simulink model "BallastSystemArchitecture"  (R2026a)
settings: Solver=VariableStepAuto
model workspace (MAT data in the model file):
  Control_Interface = Simulink.Bus
  Control_Interface.Alignment = -1
  Control_Interface.PreserveElementDimensions = 0
  Control_Interface.Elements_internal(1) = Simulink.BusElement
  Control_Interface.Elements_internal(1).Min_internal = 0
  Control_Interface.Elements_internal(1).Max_internal = 100
  Control_Interface.Elements_internal(1).DimensionsMode = 'Fixed'
  Control_Interface.Elements_internal(1).SamplingMode = 'Sample based'
  Control_Interface.Elements_internal(1).SampleTime = -1
  Control_Interface.Elements_internal(1).DocUnits = '%'
  Control_Interface.Elements_internal(1).Name = 'TankLevel'
  Control_Interface.Elements_internal(1).DataType_internal = 'double'
  Control_Interface.Elements_internal(1).Complexity = 'real'
  Control_Interface.Elements_internal(1).Dimensions = 1
  Control_Interface.Elements_internal(2) = Simulink.BusElement
  Control_Interface.Elements_internal(2).Min_internal = 0
  Control_Interface.Elements_internal(2).Max_internal = 1800
  Control_Interface.Elements_internal(2).DimensionsMode = 'Fixed'
  Control_Interface.Elements_internal(2).SamplingMode = 'Sample based'
  Control_Interface.Elements_internal(2).SampleTime = -1
  Control_Interface.Elements_internal(2).DocUnits = 'rpm'
  Control_Interface.Elements_internal(2).Name = 'PumpSpeed'
  Control_Interface.Elements_internal(2).DataType_internal = 'double'
  Control_Interface.Elements_internal(2).Complexity = 'real'
  Control_Interface.Elements_internal(2).Dimensions = 1
  Control_Interface.Elements_internal(3) = Simulink.BusElement
  Control_Interface.Elements_internal(3).Min_internal = 0
  Control_Interface.Elements_internal(3).Max_internal = 1
  Control_Interface.Elements_internal(3).DimensionsMode = 'Fixed'
  Control_Interface.Elements_internal(3).SamplingMode = 'Sample based'
  Control_Interface.Elements_internal(3).SampleTime = -1
  Control_Interface.Elements_internal(3).Name = 'ValveCommand'
  Control_Interface.Elements_internal(3).DataType_internal = 'boolean'
  Control_Interface.Elements_internal(3).Complexity = 'real'
  Control_Interface.Elements_internal(3).Dimensions = 1
  Control_Interface.DataScope = 'Auto'
  Electrical_Interface = Simulink.Bus
  Electrical_Interface.Alignment = -1
  Electrical_Interface.PreserveElementDimensions = 0
  Electrical_Interface.Elements_internal(1) = Simulink.BusElement
  Electrical_Interface.Elements_internal(1).Min_internal = 0
  Electrical_Interface.Elements_internal(1).Max_internal = 135
  Electrical_Interface.Elements_internal(1).DimensionsMode = 'Fixed'
  Electrical_Interface.Elements_internal(1).SamplingMode = 'Sample based'
  Electrical_Interface.Elements_internal(1).SampleTime = -1
  Electrical_Interface.Elements_internal(1).DocUnits = 'hp'
  Electrical_Interface.Elements_internal(1).Name = 'PowerDemand'
  Electrical_Interface.Elements_internal(1).DataType_internal = 'double'
  Electrical_Interface.Elements_internal(1).Complexity = 'real'
  Electrical_Interface.Elements_internal(1).Dimensions = 1
  Electrical_Interface.Elements_internal(2) = Simulink.BusElement
  Electrical_Interface.Elements_internal(2).Min_internal = 0
  Electrical_Interface.Elements_internal(2).Max_internal = 150
  Electrical_Interface.Elements_internal(2).DimensionsMode = 'Fixed'
  Electrical_Interface.Elements_internal(2).SamplingMode = 'Sample based'
  Electrical_Interface.Elements_internal(2).SampleTime = -1
  Electrical_Interface.Elements_internal(2).DocUnits = 'A'
  Electrical_Interface.Elements_internal(2).Name = 'Current'
  Electrical_Interface.Elements_internal(2).DataType_internal = 'double'
  Electrical_Interface.Elements_internal(2).Complexity = 'real'
  Electrical_Interface.Elements_internal(2).Dimensions = 1
  Electrical_Interface.Elements_internal(3) = Simulink.BusElement
  Electrical_Interface.Elements_internal(3).Min_internal = 0
  Electrical_Interface.Elements_internal(3).Max_internal = 480
  Electrical_Interface.Elements_internal(3).DimensionsMode = 'Fixed'
  Electrical_Interface.Elements_internal(3).SamplingMode = 'Sample based'
  Electrical_Interface.Elements_internal(3).SampleTime = -1
  Electrical_Interface.Elements_internal(3).DocUnits = 'V'
  Electrical_Interface.Elements_internal(3).Name = 'Voltage'
  Electrical_Interface.Elements_internal(3).DataType_internal = 'double'
  Electrical_Interface.Elements_internal(3).Complexity = 'real'
  Electrical_Interface.Elements_internal(3).Dimensions = 1
  Electrical_Interface.DataScope = 'Auto'
  Fluid_Interface = Simulink.Bus
  Fluid_Interface.Alignment = -1
  Fluid_Interface.PreserveElementDimensions = 0
  Fluid_Interface.Elements_internal(1) = Simulink.BusElement
  Fluid_Interface.Elements_internal(1).Min_internal = 0
  Fluid_Interface.Elements_internal(1).Max_internal = 150
  Fluid_Interface.Elements_internal(1).DimensionsMode = 'Fixed'
  Fluid_Interface.Elements_internal(1).SamplingMode = 'Sample based'
  Fluid_Interface.Elements_internal(1).SampleTime = -1
  Fluid_Interface.Elements_internal(1).DocUnits = 'psi'
  Fluid_Interface.Elements_internal(1).Name = 'Pressure'
  Fluid_Interface.Elements_internal(1).DataType_internal = 'double'
  Fluid_Interface.Elements_internal(1).Complexity = 'real'
  Fluid_Interface.Elements_internal(1).Dimensions = 1
  Fluid_Interface.Elements_internal(2) = Simulink.BusElement
  Fluid_Interface.Elements_internal(2).Min_internal = 0
  Fluid_Interface.Elements_internal(2).Max_internal = 5000
  Fluid_Interface.Elements_internal(2).DimensionsMode = 'Fixed'
  Fluid_Interface.Elements_internal(2).SamplingMode = 'Sample based'
  Fluid_Interface.Elements_internal(2).SampleTime = -1
  Fluid_Interface.Elements_internal(2).DocUnits = 'gal/hr'
  Fluid_Interface.Elements_internal(2).Name = 'FlowRate'
  Fluid_Interface.Elements_internal(2).DataType_internal = 'double'
  Fluid_Interface.Elements_internal(2).Complexity = 'real'
  Fluid_Interface.Elements_internal(2).Dimensions = 1
  Fluid_Interface.DataScope = 'Auto'
settings Model: Creator=KKoch28  LastModifiedBy=KKoch28

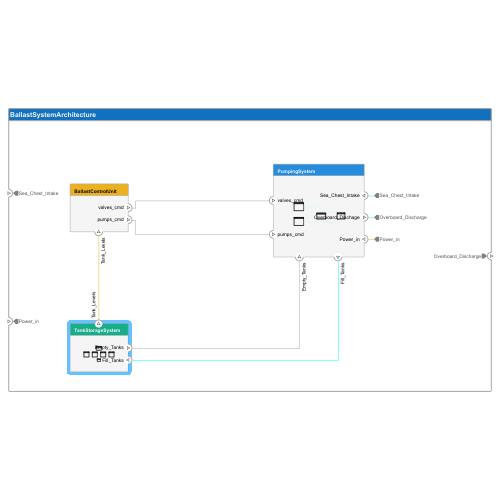
[thumbnail: Simulink's stored preview of the top-level diagram]
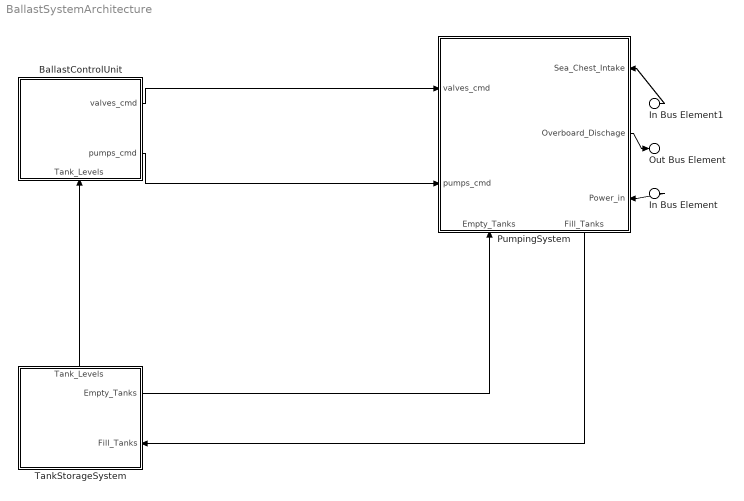
== system BallastSystemArchitecture ==
  In Bus Element1 : Inport  PortName=Sea_Chest_Intake
  In Bus Element : Inport  Port=2  PortName=Power_in
  BallastControlUnit : Subsystem
      settings: PortSchema="{\"entries\":[{\"content\":{\"headerSize\":26,\"margin\":15,\"minimumSpacing\":25,\"sides\":[{\"content\":{},\"type\":\"ConnectorPlacement.EquallySpacedRectSide\",\"uuid\":\"7b48e5ab-cef8-46bf-b1bf-123f01b56f06\"},{\"content\":{\"connectorIds\":[\"Out1\",\"Out2\"],\"side\":\"RIGHT\"},\"type\":\"ConnectorPlacement.EquallySpacedRectSide\",\"uuid\":\"927bafbe-1cb8-4d60-bc20-a78fbfb89dce\"},{\"content\":{\"side\":\"TOP\"},\"type\":\"ConnectorPlacement.EquallySpacedRectSide\",\"uuid\":\"6ef058e5-8005-46e3-bc6d-037462f0e4a9\"},{\"content\":{\"connectorIds\":[\"In1\"],\"side\":\"BOTTOM\"},\"type\":\"ConnectorPlacement.EquallySpacedRectSide\",\"uuid\":\"8c71177b-847f-47fd-b339-2dc1565e42d7\"}]},\"type\":\"ConnectorPlacement.EquallySpacedConnector\",\"uuid\":\"76570077-6843-407e-8a7f-bb3f1fbcb72b\"}],\"packageUris\":[\"http://schema.mathworks.com/mf0/Connector/R2020b\"],\"version\":\"1.0\"}"
  PumpingSystem : Subsystem
      settings: PortSchema="{\"entries\":[{\"content\":{\"headerSize\":26,\"margin\":15,\"minimumSpacing\":25,\"sides\":[{\"content\":{\"connectorIds\":[\"In4\",\"In5\"]},\"type\":\"ConnectorPlacement.EquallySpacedRectSide\",\"uuid\":\"7b48e5ab-cef8-46bf-b1bf-123f01b56f06\"},{\"content\":{\"connectorIds\":[\"In2\",\"Out1\",\"In3\"],\"side\":\"RIGHT\"},\"type\":\"ConnectorPlacement.EquallySpacedRectSide\",\"uuid\":\"927bafbe-1cb8-4d60-bc20-a78fbfb89dce\"},{\"content\":{\"side\":\"TOP\"},\"type\":\"ConnectorPlacement.EquallySpacedRectSide\",\"uuid\":\"6ef058e5-8005-46e3-bc6d-037462f0e4a9\"},{\"content\":{\"connectorIds\":[\"In1\",\"Out2\"],\"side\":\"BOTTOM\"},\"type\":\"ConnectorPlacement.EquallySpacedRectSide\",\"uuid\":\"f8b40303-dcc1-45cb-a122-b0f5fa5ded78\"}]},\"type\":\"ConnectorPlacement.EquallySpacedConnector\",\"uuid\":\"76570077-6843-407e-8a7f-bb3f1fbcb72b\"}],\"packageUris\":[\"http://schema.mathworks.com/mf0/Connector/R2020b\"],\"version\":\"1.0\"}"
  TankStorageSystem : Subsystem
      settings: PortSchema="{\"entries\":[{\"content\":{\"headerSize\":26,\"margin\":15,\"minimumSpacing\":25,\"sides\":[{\"content\":{},\"type\":\"ConnectorPlacement.EquallySpacedRectSide\",\"uuid\":\"7b48e5ab-cef8-46bf-b1bf-123f01b56f06\"},{\"content\":{\"connectorIds\":[\"Out1\",\"In1\"],\"side\":\"RIGHT\"},\"type\":\"ConnectorPlacement.EquallySpacedRectSide\",\"uuid\":\"927bafbe-1cb8-4d60-bc20-a78fbfb89dce\"},{\"content\":{\"connectorIds\":[\"Out2\"],\"side\":\"TOP\"},\"type\":\"ConnectorPlacement.EquallySpacedRectSide\",\"uuid\":\"6ef058e5-8005-46e3-bc6d-037462f0e4a9\"}]},\"type\":\"ConnectorPlacement.EquallySpacedConnector\",\"uuid\":\"76570077-6843-407e-8a7f-bb3f1fbcb72b\"}],\"packageUris\":[\"http://schema.mathworks.com/mf0/Connector/R2020b\"],\"version\":\"1.0\"}"
  Out Bus Element : Outport  PortName=Overboard_Discharge
  wires:
  BallastControlUnit/1(valves_cmd) -> PumpingSystem/4(valves_cmd)
  BallastControlUnit/2(pumps_cmd) -> PumpingSystem/5(pumps_cmd)
  TankStorageSystem/2(Tank_Levels) -> BallastControlUnit/1(Tank_Levels)
  In Bus Element/1 -> PumpingSystem/3(Power_in)
  PumpingSystem/2(Fill_Tanks) -> TankStorageSystem/1(Fill_Tanks)
  In Bus Element1/1 -> PumpingSystem/2(Sea_Chest_Intake)
  PumpingSystem/1(Overboard_Dischage) -> Out Bus Element/1
  TankStorageSystem/1(Empty_Tanks) -> PumpingSystem/1(Empty_Tanks)

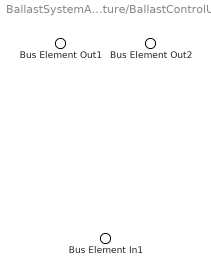
== system BallastSystemArchitecture/BallastControlUnit ==
  Bus Element In1 : Inport  PortName=Tank_Levels
  Bus Element Out1 : Outport  PortName=valves_cmd
  Bus Element Out2 : Outport  Port=2  PortName=pumps_cmd

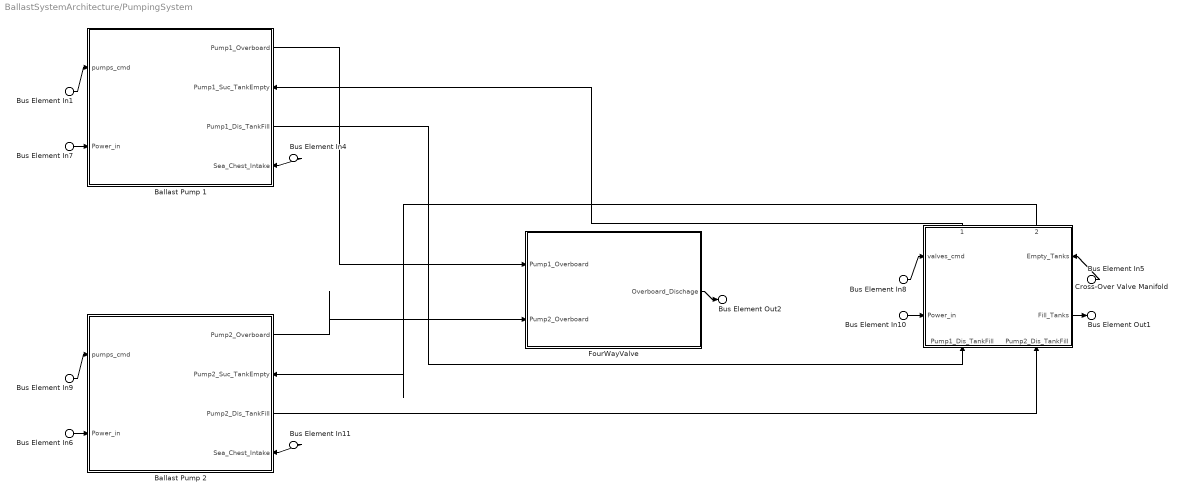
== system BallastSystemArchitecture/PumpingSystem ==
  Bus Element In5 : Inport  PortName=Empty_Tanks
  Bus Element In4 : Inport  Port=2  PortName=Sea_Chest_Intake
  Bus Element In11 : Inport  Port=2  PortName=Sea_Chest_Intake
  Bus Element In6 : Inport  Port=3  PortName=Power_in
  Bus Element In7 : Inport  Port=3  PortName=Power_in
  Bus Element In10 : Inport  Port=3  PortName=Power_in
  Bus Element In8 : Inport  Port=4  PortName=valves_cmd
  Bus Element In1 : Inport  Port=5  PortName=pumps_cmd
  Bus Element In9 : Inport  Port=5  PortName=pumps_cmd
  Ballast Pump 1 : Subsystem
      settings: PortSchema="{\"entries\":[{\"content\":{\"headerSize\":26,\"margin\":15,\"minimumSpacing\":25,\"sides\":[{\"content\":{\"connectorIds\":[\"In3\",\"In4\"]},\"type\":\"ConnectorPlacement.EquallySpacedRectSide\",\"uuid\":\"7b48e5ab-cef8-46bf-b1bf-123f01b56f06\"},{\"content\":{\"connectorIds\":[\"Out1\",\"In1\",\"Out2\",\"In2\"],\"side\":\"RIGHT\"},\"type\":\"ConnectorPlacement.EquallySpacedRectSide\",\"uuid\":\"927bafbe-1cb8-4d60-bc20-a78fbfb89dce\"},{\"content\":{\"side\":\"TOP\"},\"type\":\"ConnectorPlacement.EquallySpacedRectSide\",\"uuid\":\"6ef058e5-8005-46e3-bc6d-037462f0e4a9\"}]},\"type\":\"ConnectorPlacement.EquallySpacedConnector\",\"uuid\":\"76570077-6843-407e-8a7f-bb3f1fbcb72b\"}],\"packageUris\":[\"http://schema.mathworks.com/mf0/Connector/R2020b\"],\"version\":\"1.0\"}"
  Ballast Pump 2 : Subsystem
      settings: PortSchema="{\"entries\":[{\"content\":{\"headerSize\":26,\"margin\":15,\"minimumSpacing\":25,\"sides\":[{\"content\":{\"connectorIds\":[\"In3\",\"In4\"]},\"type\":\"ConnectorPlacement.EquallySpacedRectSide\",\"uuid\":\"7b48e5ab-cef8-46bf-b1bf-123f01b56f06\"},{\"content\":{\"connectorIds\":[\"Out1\",\"In1\",\"Out2\",\"In2\"],\"side\":\"RIGHT\"},\"type\":\"ConnectorPlacement.EquallySpacedRectSide\",\"uuid\":\"927bafbe-1cb8-4d60-bc20-a78fbfb89dce\"},{\"content\":{\"side\":\"TOP\"},\"type\":\"ConnectorPlacement.EquallySpacedRectSide\",\"uuid\":\"6ef058e5-8005-46e3-bc6d-037462f0e4a9\"}]},\"type\":\"ConnectorPlacement.EquallySpacedConnector\",\"uuid\":\"76570077-6843-407e-8a7f-bb3f1fbcb72b\"}],\"packageUris\":[\"http://schema.mathworks.com/mf0/Connector/R2020b\"],\"version\":\"1.0\"}"
  Cross-Over Valve Manifold : Subsystem
      settings: PortSchema="{\"entries\":[{\"content\":{\"headerSize\":26,\"margin\":15,\"minimumSpacing\":25,\"sides\":[{\"content\":{\"connectorIds\":[\"In4\",\"In5\"]},\"type\":\"ConnectorPlacement.EquallySpacedRectSide\",\"uuid\":\"7b48e5ab-cef8-46bf-b1bf-123f01b56f06\"},{\"content\":{\"connectorIds\":[\"In1\",\"Out3\"],\"side\":\"RIGHT\"},\"type\":\"ConnectorPlacement.EquallySpacedRectSide\",\"uuid\":\"927bafbe-1cb8-4d60-bc20-a78fbfb89dce\"},{\"content\":{\"connectorIds\":[\"Out1\",\"Out2\"],\"side\":\"TOP\"},\"type\":\"ConnectorPlacement.EquallySpacedRectSide\",\"uuid\":\"6ef058e5-8005-46e3-bc6d-037462f0e4a9\"},{\"content\":{\"connectorIds\":[\"In2\",\"In3\"],\"side\":\"BOTTOM\"},\"type\":\"ConnectorPlacement.EquallySpacedRectSide\",\"uuid\":\"57f20b38-4afd-47d2-908e-8eb658c224b8\"}]},\"type\":\"ConnectorPlacement.EquallySpacedConnector\",\"uuid\":\"76570077-6843-407e-8a7f-bb3f1fbcb72b\"}],\"packageUris\":[\"http://schema.mathworks.com/mf0/Connector/R2020b\"],\"version\":\"1.0\"}"
  FourWayValve : Subsystem
      settings: PortSchema="{\"entries\":[{\"content\":{\"headerSize\":26,\"margin\":15,\"minimumSpacing\":25,\"sides\":[{\"content\":{\"connectorIds\":[\"In1\",\"In2\"]},\"type\":\"ConnectorPlacement.EquallySpacedRectSide\",\"uuid\":\"7b48e5ab-cef8-46bf-b1bf-123f01b56f06\"},{\"content\":{\"connectorIds\":[\"Out1\"],\"side\":\"RIGHT\"},\"type\":\"ConnectorPlacement.EquallySpacedRectSide\",\"uuid\":\"927bafbe-1cb8-4d60-bc20-a78fbfb89dce\"},{\"content\":{\"side\":\"TOP\"},\"type\":\"ConnectorPlacement.EquallySpacedRectSide\",\"uuid\":\"6ef058e5-8005-46e3-bc6d-037462f0e4a9\"}]},\"type\":\"ConnectorPlacement.EquallySpacedConnector\",\"uuid\":\"76570077-6843-407e-8a7f-bb3f1fbcb72b\"}],\"packageUris\":[\"http://schema.mathworks.com/mf0/Connector/R2020b\"],\"version\":\"1.0\"}"
  Bus Element Out2 : Outport  PortName=Overboard_Dischage
  Bus Element Out1 : Outport  Port=2  PortName=Fill_Tanks
  wires:
  Bus Element In6/1 -> Ballast Pump 2/4(Power_in)
  Bus Element In7/1 -> Ballast Pump 1/4(Power_in)
  Bus Element In1/1 -> Ballast Pump 1/3(pumps_cmd)
  Bus Element In8/1 -> Cross-Over Valve Manifold/4(valves_cmd)
  Bus Element In9/1 -> Ballast Pump 2/3(pumps_cmd)
  Bus Element In10/1 -> Cross-Over Valve Manifold/5(Power_in)
  Bus Element In4/1 -> Ballast Pump 1/2(Sea_Chest_Intake)
  Bus Element In11/1 -> Ballast Pump 2/2(Sea_Chest_Intake)
  Cross-Over Valve Manifold/3(Fill_Tanks) -> Bus Element Out1/1
  Bus Element In5/1 -> Cross-Over Valve Manifold/1(Empty_Tanks)
  FourWayValve/1(Overboard_Dischage) -> Bus Element Out2/1
  Ballast Pump 1/1(Pump1_Overboard) -> FourWayValve/1(Pump1_Overboard)
  Ballast Pump 2/1(Pump2_Overboard) -> FourWayValve/2(Pump2_Overboard)
  Cross-Over Valve Manifold/1(Pump1_Suc_TankEmpty) -> Ballast Pump 1/1(Pump1_Suc_TankEmpty)
  Cross-Over Valve Manifold/2(Pump2_Suc_TankEmpty) -> Ballast Pump 2/1(Pump2_Suc_TankEmpty)
  Ballast Pump 2/2(Pump2_Dis_TankFill) -> Cross-Over Valve Manifold/3(Pump2_Dis_TankFill)
  Ballast Pump 1/2(Pump1_Dis_TankFill) -> Cross-Over Valve Manifold/2(Pump1_Dis_TankFill)

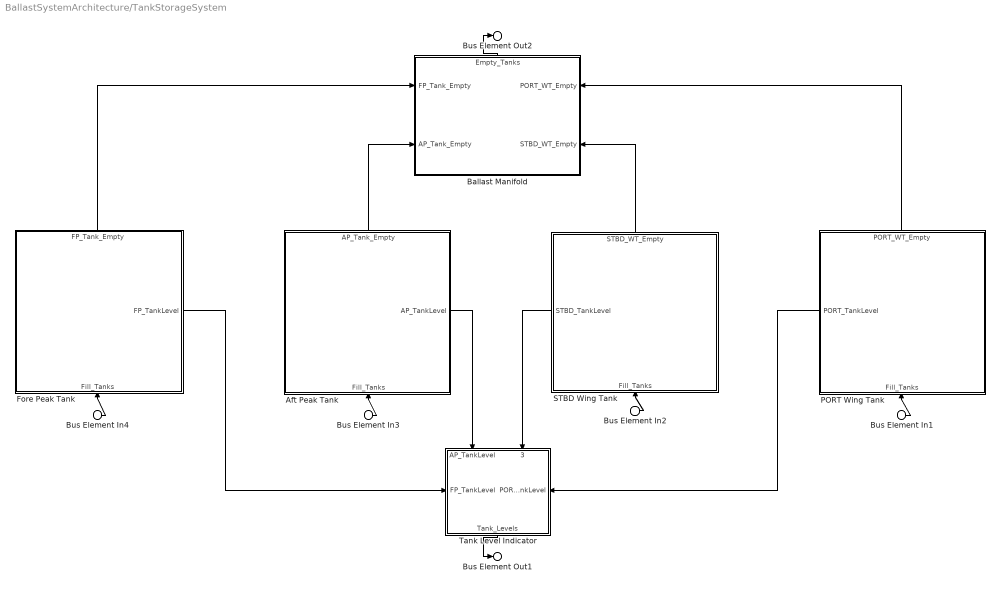
== system BallastSystemArchitecture/TankStorageSystem ==
  Bus Element In{1..4} (4 alike) : Inport  PortName=Fill_Tanks
  Aft Peak Tank : Subsystem
      settings: PortSchema="{\"entries\":[{\"content\":{\"headerSize\":26,\"margin\":15,\"minimumSpacing\":25,\"sides\":[{\"content\":{},\"type\":\"ConnectorPlacement.EquallySpacedRectSide\",\"uuid\":\"7b48e5ab-cef8-46bf-b1bf-123f01b56f06\"},{\"content\":{\"connectorIds\":[\"Out1\"],\"side\":\"RIGHT\"},\"type\":\"ConnectorPlacement.EquallySpacedRectSide\",\"uuid\":\"927bafbe-1cb8-4d60-bc20-a78fbfb89dce\"},{\"content\":{\"connectorIds\":[\"Out2\"],\"side\":\"TOP\"},\"type\":\"ConnectorPlacement.EquallySpacedRectSide\",\"uuid\":\"6ef058e5-8005-46e3-bc6d-037462f0e4a9\"},{\"content\":{\"connectorIds\":[\"In1\"],\"side\":\"BOTTOM\"},\"type\":\"ConnectorPlacement.EquallySpacedRectSide\",\"uuid\":\"b0a68243-15d1-455e-9233-3eeab8319efc\"}]},\"type\":\"ConnectorPlacement.EquallySpacedConnector\",\"uuid\":\"76570077-6843-407e-8a7f-bb3f1fbcb72b\"}],\"packageUris\":[\"http://schema.mathworks.com/mf0/Connector/R2020b\"],\"version\":\"1.0\"}"
  Ballast Manifold : Subsystem
      settings: PortSchema="{\"entries\":[{\"content\":{\"headerSize\":26,\"margin\":15,\"minimumSpacing\":25,\"sides\":[{\"content\":{\"connectorIds\":[\"In3\",\"In4\"]},\"type\":\"ConnectorPlacement.EquallySpacedRectSide\",\"uuid\":\"7caacf18-7747-4ecc-af71-45c03ac2bed9\"},{\"content\":{\"connectorIds\":[\"In1\",\"In2\"],\"side\":\"RIGHT\"},\"type\":\"ConnectorPlacement.EquallySpacedRectSide\",\"uuid\":\"e5805487-b9d8-4e83-8787-126e62b1bebe\"},{\"content\":{\"connectorIds\":[\"Out1\"],\"side\":\"TOP\"},\"type\":\"ConnectorPlacement.EquallySpacedRectSide\",\"uuid\":\"1e00032c-6755-472f-be9b-472f5548cbb0\"}]},\"type\":\"ConnectorPlacement.EquallySpacedConnector\",\"uuid\":\"baf99c29-53a6-4539-8317-941f1430e3b9\"}],\"packageUris\":[\"http://schema.mathworks.com/mf0/Connector/R2020b\"],\"version\":\"1.0\"}"
  Fore Peak Tank : Subsystem
      settings: PortSchema="{\"entries\":[{\"content\":{\"headerSize\":26,\"margin\":15,\"minimumSpacing\":25,\"sides\":[{\"content\":{},\"type\":\"ConnectorPlacement.EquallySpacedRectSide\",\"uuid\":\"7b48e5ab-cef8-46bf-b1bf-123f01b56f06\"},{\"content\":{\"connectorIds\":[\"Out1\"],\"side\":\"RIGHT\"},\"type\":\"ConnectorPlacement.EquallySpacedRectSide\",\"uuid\":\"927bafbe-1cb8-4d60-bc20-a78fbfb89dce\"},{\"content\":{\"connectorIds\":[\"Out2\"],\"side\":\"TOP\"},\"type\":\"ConnectorPlacement.EquallySpacedRectSide\",\"uuid\":\"6ef058e5-8005-46e3-bc6d-037462f0e4a9\"},{\"content\":{\"connectorIds\":[\"In1\"],\"side\":\"BOTTOM\"},\"type\":\"ConnectorPlacement.EquallySpacedRectSide\",\"uuid\":\"2c10b5a3-8f2c-49c7-bc02-293140a2a56d\"}]},\"type\":\"ConnectorPlacement.EquallySpacedConnector\",\"uuid\":\"76570077-6843-407e-8a7f-bb3f1fbcb72b\"}],\"packageUris\":[\"http://schema.mathworks.com/mf0/Connector/R2020b\"],\"version\":\"1.0\"}"
  PORT Wing Tank : Subsystem
      settings: PortSchema="{\"entries\":[{\"content\":{\"headerSize\":26,\"margin\":15,\"minimumSpacing\":25,\"sides\":[{\"content\":{\"connectorIds\":[\"Out1\"]},\"type\":\"ConnectorPlacement.EquallySpacedRectSide\",\"uuid\":\"7b48e5ab-cef8-46bf-b1bf-123f01b56f06\"},{\"content\":{\"side\":\"RIGHT\"},\"type\":\"ConnectorPlacement.EquallySpacedRectSide\",\"uuid\":\"927bafbe-1cb8-4d60-bc20-a78fbfb89dce\"},{\"content\":{\"connectorIds\":[\"Out2\"],\"side\":\"TOP\"},\"type\":\"ConnectorPlacement.EquallySpacedRectSide\",\"uuid\":\"6ef058e5-8005-46e3-bc6d-037462f0e4a9\"},{\"content\":{\"connectorIds\":[\"In1\"],\"side\":\"BOTTOM\"},\"type\":\"ConnectorPlacement.EquallySpacedRectSide\",\"uuid\":\"f0ab6ee1-62ad-4ec5-bea4-b04d656e17c5\"}]},\"type\":\"ConnectorPlacement.EquallySpacedConnector\",\"uuid\":\"76570077-6843-407e-8a7f-bb3f1fbcb72b\"}],\"packageUris\":[\"http://schema.mathworks.com/mf0/Connector/R2020b\"],\"version\":\"1.0\"}"
  STBD Wing Tank : Subsystem
      settings: PortSchema="{\"entries\":[{\"content\":{\"headerSize\":26,\"margin\":15,\"minimumSpacing\":25,\"sides\":[{\"content\":{\"connectorIds\":[\"Out1\"]},\"type\":\"ConnectorPlacement.EquallySpacedRectSide\",\"uuid\":\"7b48e5ab-cef8-46bf-b1bf-123f01b56f06\"},{\"content\":{\"side\":\"RIGHT\"},\"type\":\"ConnectorPlacement.EquallySpacedRectSide\",\"uuid\":\"927bafbe-1cb8-4d60-bc20-a78fbfb89dce\"},{\"content\":{\"connectorIds\":[\"Out2\"],\"side\":\"TOP\"},\"type\":\"ConnectorPlacement.EquallySpacedRectSide\",\"uuid\":\"6ef058e5-8005-46e3-bc6d-037462f0e4a9\"},{\"content\":{\"connectorIds\":[\"In1\"],\"side\":\"BOTTOM\"},\"type\":\"ConnectorPlacement.EquallySpacedRectSide\",\"uuid\":\"567913fe-02f7-4cb7-8814-8023e1ed5525\"}]},\"type\":\"ConnectorPlacement.EquallySpacedConnector\",\"uuid\":\"76570077-6843-407e-8a7f-bb3f1fbcb72b\"}],\"packageUris\":[\"http://schema.mathworks.com/mf0/Connector/R2020b\"],\"version\":\"1.0\"}"
  Tank Level Indicator : Subsystem
      settings: PortSchema="{\"entries\":[{\"content\":{\"headerSize\":26,\"margin\":15,\"minimumSpacing\":25,\"sides\":[{\"content\":{\"connectorIds\":[\"In2\"]},\"type\":\"ConnectorPlacement.EquallySpacedRectSide\",\"uuid\":\"7caacf18-7747-4ecc-af71-45c03ac2bed9\"},{\"content\":{\"connectorIds\":[\"In1\"],\"side\":\"RIGHT\"},\"type\":\"ConnectorPlacement.EquallySpacedRectSide\",\"uuid\":\"e5805487-b9d8-4e83-8787-126e62b1bebe\"},{\"content\":{\"connectorIds\":[\"In4\",\"In3\"],\"side\":\"TOP\"},\"type\":\"ConnectorPlacement.EquallySpacedRectSide\",\"uuid\":\"1e00032c-6755-472f-be9b-472f5548cbb0\"},{\"content\":{\"connectorIds\":[\"Out1\"],\"side\":\"BOTTOM\"},\"type\":\"ConnectorPlacement.EquallySpacedRectSide\",\"uuid\":\"95ff12c5-cc2f-4212-bab3-b4a2fafa697d\"}]},\"type\":\"ConnectorPlacement.EquallySpacedConnector\",\"uuid\":\"baf99c29-53a6-4539-8317-941f1430e3b9\"}],\"packageUris\":[\"http://schema.mathworks.com/mf0/Connector/R2020b\"],\"version\":\"1.0\"}"
  Bus Element Out2 : Outport  PortName=Empty_Tanks
  Bus Element Out1 : Outport  Port=2  PortName=Tank_Levels
  wires:
  Bus Element In1/1 -> PORT Wing Tank/1(Fill_Tanks)
  Bus Element In2/1 -> STBD Wing Tank/1(Fill_Tanks)
  Bus Element In3/1 -> Aft Peak Tank/1(Fill_Tanks)
  Bus Element In4/1 -> Fore Peak Tank/1(Fill_Tanks)
  Fore Peak Tank/2(FP_Tank_Empty) -> Ballast Manifold/3(FP_Tank_Empty)
  Aft Peak Tank/2(AP_Tank_Empty) -> Ballast Manifold/4(AP_Tank_Empty)
  STBD Wing Tank/2(STBD_WT_Empty) -> Ballast Manifold/2(STBD_WT_Empty)
  PORT Wing Tank/2(PORT_WT_Empty) -> Ballast Manifold/1(PORT_WT_Empty)
  Ballast Manifold/1(Empty_Tanks) -> Bus Element Out2/1
  Aft Peak Tank/1(AP_TankLevel) -> Tank Level Indicator/4(AP_TankLevel)
  Fore Peak Tank/1(FP_TankLevel) -> Tank Level Indicator/2(FP_TankLevel)
  STBD Wing Tank/1(STBD_TankLevel) -> Tank Level Indicator/3(STBD_TankLevel)
  PORT Wing Tank/1(PORT_TankLevel) -> Tank Level Indicator/1(PORT_TankLevel)
  Tank Level Indicator/1(Tank_Levels) -> Bus Element Out1/1

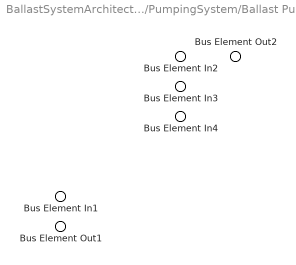
== system BallastSystemArchitecture/PumpingSystem/Ballast Pump 1 ==
  Bus Element In4 : Inport  PortName=Pump1_Suc_TankEmpty
  Bus Element In3 : Inport  Port=2  PortName=Sea_Chest_Intake
  Bus Element In2 : Inport  Port=3  PortName=pumps_cmd
  Bus Element In1 : Inport  Port=4  PortName=Power_in
  Bus Element Out2 : Outport  PortName=Pump1_Overboard
  Bus Element Out1 : Outport  Port=2  PortName=Pump1_Dis_TankFill

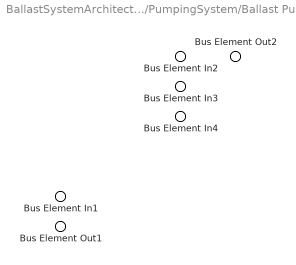
== system BallastSystemArchitecture/PumpingSystem/Ballast Pump 2 ==
  Bus Element In4 : Inport  PortName=Pump2_Suc_TankEmpty
  Bus Element In3 : Inport  Port=2  PortName=Sea_Chest_Intake
  Bus Element In2 : Inport  Port=3  PortName=pumps_cmd
  Bus Element In1 : Inport  Port=4  PortName=Power_in
  Bus Element Out2 : Outport  PortName=Pump2_Overboard
  Bus Element Out1 : Outport  Port=2  PortName=Pump2_Dis_TankFill

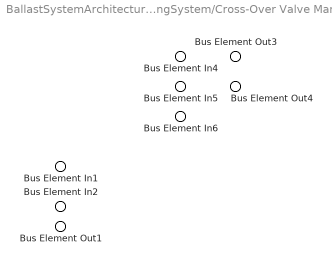
== system BallastSystemArchitecture/PumpingSystem/Cross-Over Valve Manifold ==
  Bus Element In6 : Inport  PortName=Empty_Tanks
  Bus Element In5 : Inport  Port=2  PortName=Pump1_Dis_TankFill
  Bus Element In4 : Inport  Port=3  PortName=Pump2_Dis_TankFill
  Bus Element In1 : Inport  Port=4  PortName=valves_cmd
  Bus Element In2 : Inport  Port=5  PortName=Power_in
  Bus Element Out4 : Outport  PortName=Pump1_Suc_TankEmpty
  Bus Element Out3 : Outport  Port=2  PortName=Pump2_Suc_TankEmpty
  Bus Element Out1 : Outport  Port=3  PortName=Fill_Tanks

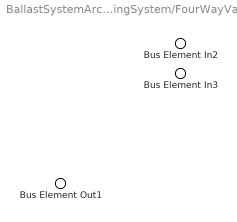
== system BallastSystemArchitecture/PumpingSystem/FourWayValve ==
  Bus Element In3 : Inport  PortName=Pump1_Overboard
  Bus Element In2 : Inport  Port=2  PortName=Pump2_Overboard
  Bus Element Out1 : Outport  PortName=Overboard_Dischage

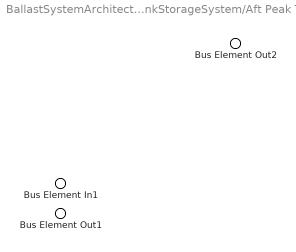
== system BallastSystemArchitecture/TankStorageSystem/Aft Peak Tank ==
  Bus Element In1 : Inport  PortName=Fill_Tanks
  Bus Element Out2 : Outport  PortName=AP_TankLevel
  Bus Element Out1 : Outport  Port=2  PortName=AP_Tank_Empty

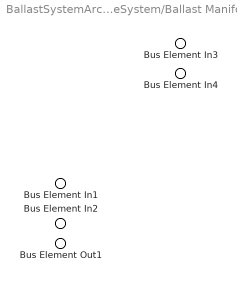
== system BallastSystemArchitecture/TankStorageSystem/Ballast Manifold ==
  Bus Element In4 : Inport  PortName=PORT_WT_Empty
  Bus Element In3 : Inport  Port=2  PortName=STBD_WT_Empty
  Bus Element In1 : Inport  Port=3  PortName=FP_Tank_Empty
  Bus Element In2 : Inport  Port=4  PortName=AP_Tank_Empty
  Bus Element Out1 : Outport  PortName=Empty_Tanks

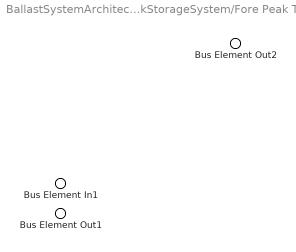
== system BallastSystemArchitecture/TankStorageSystem/Fore Peak Tank ==
  Bus Element In1 : Inport  PortName=Fill_Tanks
  Bus Element Out2 : Outport  PortName=FP_TankLevel
  Bus Element Out1 : Outport  Port=2  PortName=FP_Tank_Empty

== system BallastSystemArchitecture/TankStorageSystem/PORT Wing Tank ==
  Bus Element In1 : Inport  PortName=Fill_Tanks
  Bus Element Out2 : Outport  PortName=PORT_TankLevel
  Bus Element Out1 : Outport  Port=2  PortName=PORT_WT_Empty

== system BallastSystemArchitecture/TankStorageSystem/STBD Wing Tank ==
  Bus Element In1 : Inport  PortName=Fill_Tanks
  Bus Element Out2 : Outport  PortName=STBD_TankLevel
  Bus Element Out1 : Outport  Port=2  PortName=STBD_WT_Empty

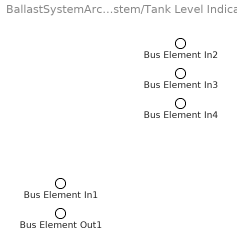
== system BallastSystemArchitecture/TankStorageSystem/Tank Level Indicator ==
  Bus Element In4 : Inport  PortName=PORT_TankLevel
  Bus Element In2 : Inport  Port=2  PortName=FP_TankLevel
  Bus Element In3 : Inport  Port=3  PortName=STBD_TankLevel
  Bus Element In1 : Inport  Port=4  PortName=AP_TankLevel
  Bus Element Out1 : Outport  PortName=Tank_Levels
